simulink model "T1DvirtualPatient"  (Simulink 10.0)
settings: Solver=ode3  StartTime=0.0  StopTime=48*60  FixedStep=dt  RelTol=1e-3  EnableMultiTasking=on
values from neighbouring files (symbols this model uses):
  dt = evalin('base','dt')    [InsulinInjection.m]    (also in MC_Simulations.m = 2; MC_Simulations_UE_OE.m = 2)
  MM = TDMC/350*EI    [MC_Simulations.m]    (also in MC_Simulations_UE_OE.m)
  x_G = x_G/x_sum    [MC_Simulations.m]    (also in MC_Simulations_UE_OE.m)
  x_P = x_P/x_sum    [MC_Simulations.m]    (also in MC_Simulations_UE_OE.m)
undefined symbols (not defined in the file or in its folder): sigbuilder_block
settings Model: Creator=Farayand  LastModifiedBy=haMed
settings DataIOCC: SignalLoggingSaveFormat=ModelDataLogs
settings OptimizationCC: ExpressionDepthLimit=2147483647
settings DebuggingCC: SolverPrmCheckMsg=warning  FcnCallInpInsideContextMsg=warning  StateNameClashWarn=warning
settings GRTTargetCC: GeneratePreprocessorConditionals=Disable all
settings ConfigComp: CovExternalEMLEnable=off  CovSFcnEnable=off
settings SimscapeCC: SimscapeNormalizeSystem=off
settings ConfigurationSet: Description=SimMechanics 2G
settings SimEventsCC: propDiagStatOutput=1  propPreventDuplicateEvents=0

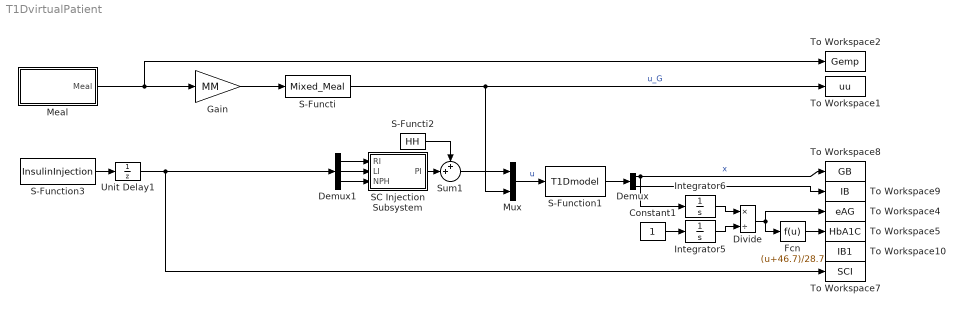
== system T1DvirtualPatient ==
  Constant1 : Constant
  Demux : Demux  Outputs=2
  Demux1 : Demux  Outputs=3
  Divide : Product  Inputs=*/
  Fcn : Fcn  Expr=(u+46.7)/28.7
  Gain : Gain  Gain=MM
  Integrator5 : Integrator
  Integrator6 : Integrator
  Meal : Subsystem  Tag=STV Subsys  LoadFcn=sigbuilder_block('load');  StartFcn=sigbuilder_block('start');  StopFcn=sigbuilder_block('stop');  ClipboardFcn=sigbuilder_block('clipboard');  mask(Sigbuilder block){tuvar=[0:10]}
      mask help: Create and generate interchangeable groups of signals whose waveforms are piecewise linear.
      mask init:
      | if ~strcmp(get_param(bdroot(gcbh),'SimulationStatus'),'stopped') tuvar = sigbuilder_block('maskInit'); end
      settings: CopyFcn=sigbuilder_block('copy');  DeleteFcn=sigbuilder_block('delete');  ModelCloseFcn=sigbuilder_block('modelClose');  PreSaveFcn=sigbuilder_block('preSave');  PauseFcn=sigbuilder_block('pause')  ContinueFcn=sigbuilder_block('continue')  NameChangeFcn=sigbuilder_block('namechange');  OpenFcn=sigbuilder_block('open',[0 22.5 1024.5 495.75 ]);  CloseFcn=sigbuilder_block('close');
      mask Display: plot(0, 0, 100, 100,[2, 2, 32, 32, 2], [68, 8, 8, 68, 68],[32, 2], [38, 38], [32, 19, 2],[53, 60, 44], [32, 17, 17, 2],[16, 16, 31, 31]);txt = getActiveGroup(gcbh);text(2, 100, txt,'verticalAlignment', 'top');
  Mux : Mux  Inputs=2
  S-Functi : S-Function  FunctionName=Mixed_Meal  Parameters=x_G,x_P,x_P  SFunctionDeploymentMode=off  EnableBusSupport=off
  S-Functi2 : S-Function  FunctionName=HH  Parameters=u_init  SFunctionDeploymentMode=off  EnableBusSupport=off
  S-Function1 : S-Function  FunctionName=T1Dmodel  Parameters=bw, age,PhysParams  SFunctionDeploymentMode=off  EnableBusSupport=off
  S-Function3 : S-Function  FunctionName=InsulinInjection  SFunctionDeploymentMode=off  EnableBusSupport=off
  SC Injection Subsystem : Subsystem
  Sum1 : Sum  Inputs=++|
  To Workspace1 : ToWorkspace  VariableName=uu  SampleTime=-1
  To Workspace10 : ToWorkspace  VariableName=IB1  SampleTime=-1
  To Workspace2 : ToWorkspace  VariableName=Gemp  SampleTime=-1
  To Workspace4 : ToWorkspace  VariableName=eAG  SampleTime=-1
  To Workspace5 : ToWorkspace  VariableName=HbA1C  SampleTime=-1
  To Workspace7 : ToWorkspace  VariableName=SCI  SampleTime=-1
  To Workspace8 : ToWorkspace  VariableName=GB  SampleTime=-1
  To Workspace9 : ToWorkspace  VariableName=IB  SampleTime=-1
  Unit Delay1 : UnitDelay  SampleTime=dt  HasFrameUpgradeWarning=on
  wires:
  Mux/1 -> S-Function1/1  "u"
  Demux/1 -> To Workspace8/1, Integrator6/1  "x"
  S-Functi/1 -> Mux/2, To Workspace1/1  "u_G"
  Constant1/1 -> Integrator5/1
  Integrator5/1 -> Divide/2
  Fcn/1 -> To Workspace5/1
  Integrator6/1 -> Divide/1
  Divide/1 -> To Workspace4/1, Fcn/1
  Meal/1(Meal) -> To Workspace2/1, Gain/1
  Demux1/1 -> SC Injection Subsystem/1(RI)
  Demux1/2 -> SC Injection Subsystem/2(LI)
  Demux1/3 -> SC Injection Subsystem/3(NPH)
  S-Function3/1 -> Unit Delay1/1
  Demux/2 -> To Workspace9/1
  Unit Delay1/1 -> Demux1/1, To Workspace7/1
  S-Function1/1 -> Demux/1
  SC Injection Subsystem/1(PI) -> Sum1/2
  Sum1/1 -> Mux/1
  S-Functi2/1 -> Sum1/1
  Gain/1 -> S-Functi/1

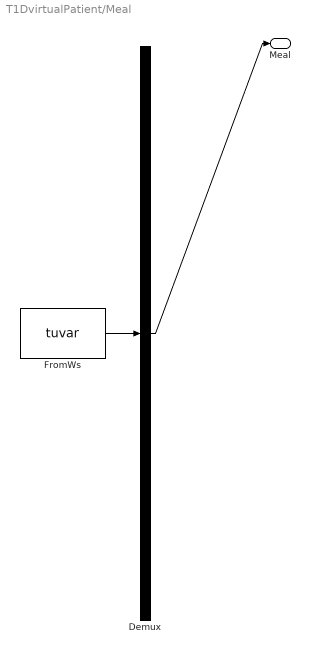
== system T1DvirtualPatient/Meal ==
  Demux : Demux  Tag=STV Demux  Outputs=1
  FromWs : FromWorkspace  Tag=STV FromWs  VariableName=tuvar  SampleTime=0  SigBuilderData=DataTag0  VnvData=DataTag1
      SigBuilderData=|
      | common.afterFinalStr = 'Extrapolate'
      | common.sampleTime = 0
      | dataSet.timeRange = [0 1333]
      | dataSet.name = 'Group 1'
      | sbobj.Groups.Name = 'Group 1'
      | sbobj.Groups.Signals.Name = 'Meal'
      | sbobj.Groups.Signals.XData = [0 30 40 80 90 180 190 200 210 330 340 380 390 570 580 590 600 810 820 845 855 1333]
      | sbobj.Groups.Signals.YData = [0 0 2 2 0 0 2 2 0 0 2 2 0 0 2 2 0 0 2 2 0 0]
      | sbobj.Groups.TimeRange = [0 1333]
  Meal : Outport  Tag=STV Outport
  wires:
  FromWs/1 -> Demux/1
  Demux/1 -> Meal/1

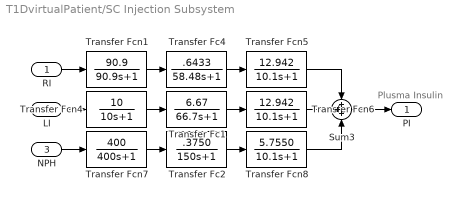
== system T1DvirtualPatient/SC Injection Subsystem ==
  note: Plusma Insulin
  RI : Inport
  LI : Inport  Port=2
  NPH : Inport  Port=3
  Sum3 : Sum  Inputs=+++
  Transfer Fc1 : TransferFcn  Numerator=[6.67]  Denominator=[66.7 1]
  Transfer Fc2 : TransferFcn  Numerator=[.3750]  Denominator=[150 1]
  Transfer Fc4 : TransferFcn  Numerator=.6433  Denominator=[58.48 1]
  Transfer Fcn1 : TransferFcn  Numerator=90.9  Denominator=[90.9 1]
  Transfer Fcn4 : TransferFcn  Numerator=[10]  Denominator=[10 1]
  Transfer Fcn5 : TransferFcn  Numerator=[12.942]  Denominator=[10.1 1]
  Transfer Fcn6 : TransferFcn  Numerator=[12.942]  Denominator=[10.1 1]
  Transfer Fcn7 : TransferFcn  Numerator=[400]  Denominator=[400 1]
  Transfer Fcn8 : TransferFcn  Numerator=[5.7550]  Denominator=[10.1 1]
  PI : Outport
  wires:
  Transfer Fcn8/1 -> Sum3/3
  Transfer Fcn6/1 -> Sum3/2
  Transfer Fcn5/1 -> Sum3/1
  Transfer Fc2/1 -> Transfer Fcn8/1
  Transfer Fcn7/1 -> Transfer Fc2/1
  Transfer Fc1/1 -> Transfer Fcn6/1
  Transfer Fcn4/1 -> Transfer Fc1/1
  Transfer Fc4/1 -> Transfer Fcn5/1
  Transfer Fcn1/1 -> Transfer Fc4/1
  RI/1 -> Transfer Fcn1/1
  Sum3/1 -> PI/1
  LI/1 -> Transfer Fcn4/1
  NPH/1 -> Transfer Fcn7/1
